simulink model "CariLQR"  (R2023b)
settings: Solver=VariableStepAuto  StartTime=0.0  StopTime=30  RelTol=1e-3
values from neighbouring files (symbols this model uses):
  A = [0 1 0 0 ... (first row only)    [FindLQR.m]    (also in GA.m)
  B = [B1 B2]    [FindLQR.m]    (also in GA.m)
  C = [0 0 1 0 ... (first row only)    [FindLQR.m]    (also in GA.m)
  K_opt = lqr(A, B, Q_opt, R_opt)    [GA.m]
undefined symbols (not defined in the file or in its folder): K_base
settings Model: Creator=izmah  LastModifiedBy=izmah
settings DebuggingCC: UnderSpecifiedDimensionMsg=error

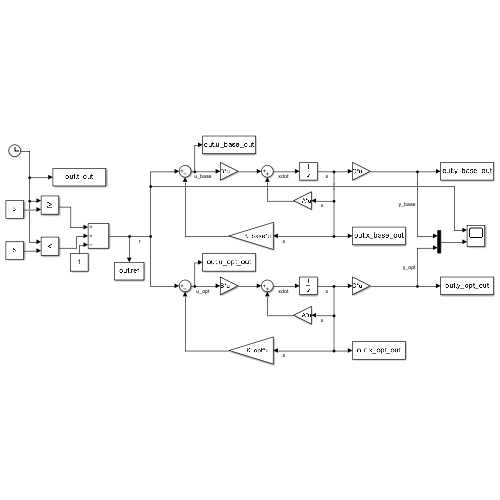
[thumbnail: Simulink's stored preview of the top-level diagram]
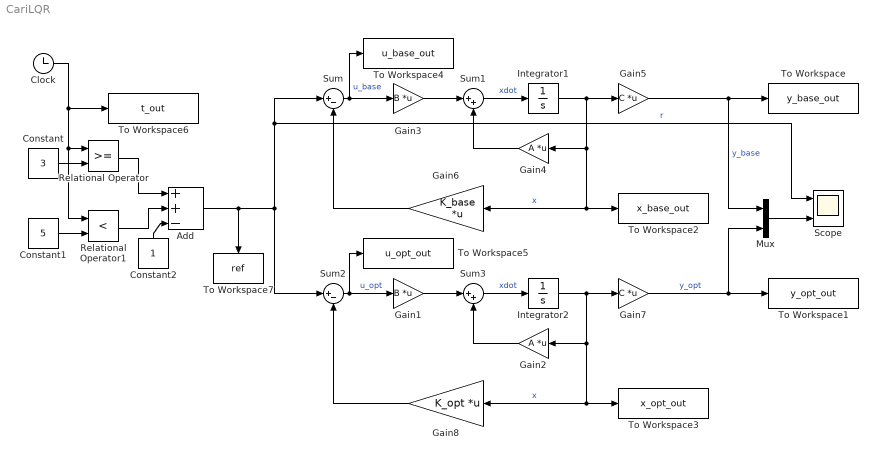
== system CariLQR ==
  Add : Sum  Inputs=++-
  Clock : Clock
  Constant : Constant  Value=3
  Constant1 : Constant  Value=5
  Constant2 : Constant
  Gain1 : Gain  Gain=B  Multiplication=Matrix(K*u)
  Gain2 : Gain  Gain=A  Multiplication=Matrix(K*u)
  Gain3 : Gain  Gain=B  Multiplication=Matrix(K*u)
  Gain4 : Gain  Gain=A  Multiplication=Matrix(K*u)
  Gain5 : Gain  Gain=C  Multiplication=Matrix(K*u)
  Gain6 : Gain  Gain=K_base  Multiplication=Matrix(K*u)
  Gain7 : Gain  Gain=C  Multiplication=Matrix(K*u)
  Gain8 : Gain  Gain=K_opt  Multiplication=Matrix(K*u)
  Integrator1 : Integrator
  Integrator2 : Integrator
  Mux : Mux  Inputs=2
  Relational Operator : RelationalOperator  OutDataTypeStr=boolean  RndMeth=Simplest  InputSameDT=off
  Relational Operator1 : RelationalOperator  Operator=<  OutDataTypeStr=boolean  RndMeth=Simplest  InputSameDT=off
  Scope : Scope  NumInputPorts=2
  Sum : Sum  Inputs=|+-
  Sum1 : Sum  Inputs=|++
  Sum2 : Sum  Inputs=|+-
  Sum3 : Sum  Inputs=|++
  To Workspace : ToWorkspace  VariableName=y_base_out  SampleTime=-1
  To Workspace1 : ToWorkspace  VariableName=y_opt_out  SampleTime=-1
  To Workspace2 : ToWorkspace  VariableName=x_base_out  SampleTime=-1
  To Workspace3 : ToWorkspace  VariableName=x_opt_out  SampleTime=-1
  To Workspace4 : ToWorkspace  VariableName=u_base_out  SampleTime=-1
  To Workspace5 : ToWorkspace  VariableName=u_opt_out  SampleTime=-1
  To Workspace6 : ToWorkspace  VariableName=t_out  SampleTime=-1
  To Workspace7 : ToWorkspace  VariableName=ref  SampleTime=-1
  wires:
  Sum1/1 -> Integrator1/1  "xdot"
  Gain3/1 -> Sum1/1
  Gain4/1 -> Sum1/2
  Integrator1/1 -> Gain5/1, Gain4/1, To Workspace2/1, Gain6/1  "x"
  Gain6/1 -> Sum/2
  Sum/1 -> Gain3/1, To Workspace4/1  "u_base"
  Gain5/1 -> To Workspace/1, Mux/1  "y_base"
  Constant/1 -> Relational Operator/2
  Constant1/1 -> Relational Operator1/2
  Clock/1 -> Relational Operator/1, Relational Operator1/1, To Workspace6/1
  Relational Operator/1 -> Add/1
  Relational Operator1/1 -> Add/2
  Constant2/1 -> Add/3
  Add/1 -> To Workspace7/1, Sum2/1, Sum/1, Scope/1  "r"
  Gain7/1 -> To Workspace1/1, Mux/2  "y_opt"
  Sum3/1 -> Integrator2/1  "xdot"
  Gain8/1 -> Sum2/2
  Sum2/1 -> Gain1/1, To Workspace5/1  "u_opt"
  Integrator2/1 -> Gain7/1, Gain2/1, To Workspace3/1, Gain8/1  "x"
  Gain2/1 -> Sum3/2
  Gain1/1 -> Sum3/1
  Mux/1 -> Scope/2
